simulink model "fanjet_simulink"  (R2015a)
settings: Solver=FixedStepDiscrete  SolverMode=SingleTasking  StartTime=0.0  StopTime=3.5  RelTol=1e-3  SampleTimeConstraint=Specified
libraries: simulink x1
settings Model: Creator=b  LastModifiedBy=jcchin
settings DataIOCC: SignalLoggingSaveFormat=ModelDataLogs
settings OptimizationCC: ExpressionDepthLimit=2147483647  InitFltsAndDblsToZero=on
settings DebuggingCC: SaveWithParameterizedLinksMsg=none  UnderspecifiedInitializationDetection=Classic  MergeDetectMultiDrivingBlocksExec=none  SignalResolutionControl=TryResolveAllWithWarning  SolverPrmCheckMsg=warning  MultiTaskDSMMsg=warning  MultiTaskCondExecSysMsg=none  FcnCallInpInsideContextMsg=EnableAllAsWarning  SFcnCompatibilityMsg=warning  StateNameClashWarn=warning
settings GRTTargetCC: TargetFcnLib=ansi_tfl_tmw.mat  CombineOutputUpdateFcns=off  GRTInterface=on

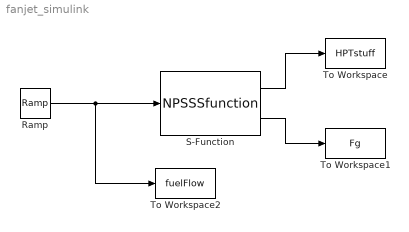
== system fanjet_simulink ==
  Ramp : simulink/Sources/Ramp  slope=.0015  start=.3  X0=.25
  S-Function : S-Function  FunctionName=NPSSSfunction  Parameters='HiBypFan.config'
  To Workspace : ToWorkspace  VariableName=HPTstuff  SampleTime=-1
  To Workspace1 : ToWorkspace  VariableName=Fg  SampleTime=-1
  To Workspace2 : ToWorkspace  VariableName=fuelFlow  SampleTime=-1
  wires:
  Ramp/1 -> To Workspace2/1, S-Function/1
  S-Function/2 -> To Workspace1/1
  S-Function/1 -> To Workspace/1
